simulink model "JointSpace_Task_v2"  (R2020b)
settings: Solver=ode3  StartTime=0.0  StopTime=6  FixedStep=0.05  RelTol=1e-3
libraries: XBotBlockToolbox x1, simulink x1, Utilities x1

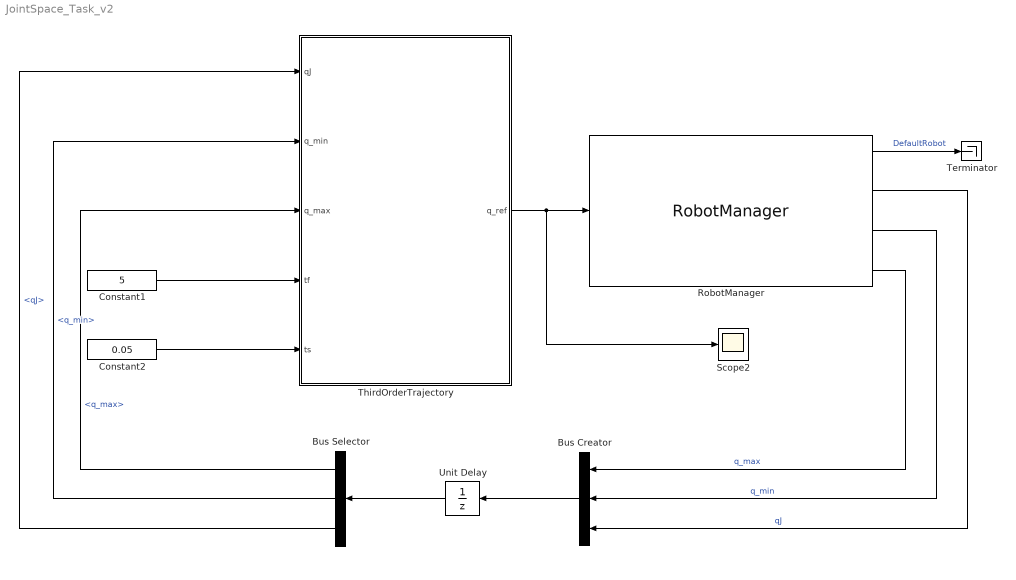
== system JointSpace_Task_v2 ==
  Bus Creator : BusCreator  Inputs=3
  Bus Selector : BusSelector  OutputSignals=q_max,q_min,qJ
  Constant1 : Constant  Value=5
  Constant2 : Constant  Value=0.05
  RobotManager : XBotBlockToolbox/RobotManager  RobotName=DefaultRobot  ModelName=DefaultModel  UseExtRobot=Off  SyncWithModel=Off  ReadingsList={ 'qJ' }  MechanicalLimitsList={ 'q_min', 'q_max' }  MechanicalLimitsCheck=Off  MechanicalLimitsEnforce=Off  SensorList={}  ReferencesList={ 'qJ_ref' }  OldRobotName=DefaultRobot
  Scope2 : Scope
  Terminator : Terminator
  ThirdOrderTrajectory : Subsystem
  Unit Delay : UnitDelay  SampleTime=-1  HasFrameUpgradeWarning=on
  wires:
  Constant1/1 -> ThirdOrderTrajectory/4(tf)
  Constant2/1 -> ThirdOrderTrajectory/5(ts)
  RobotManager/1 -> Terminator/1  "DefaultRobot"
  ThirdOrderTrajectory/1(q_ref) -> Scope2/1, RobotManager/1
  RobotManager/3 -> Bus Creator/2  "q_min"
  RobotManager/4 -> Bus Creator/1  "q_max"
  Bus Creator/1 -> Unit Delay/1
  Unit Delay/1 -> Bus Selector/1
  Bus Selector/1 -> ThirdOrderTrajectory/3(q_max)  "<q_max>"
  Bus Selector/2 -> ThirdOrderTrajectory/2(q_min)  "<q_min>"
  Bus Selector/3 -> ThirdOrderTrajectory/1(qJ)  "<qJ>"
  RobotManager/2 -> Bus Creator/3  "qJ"

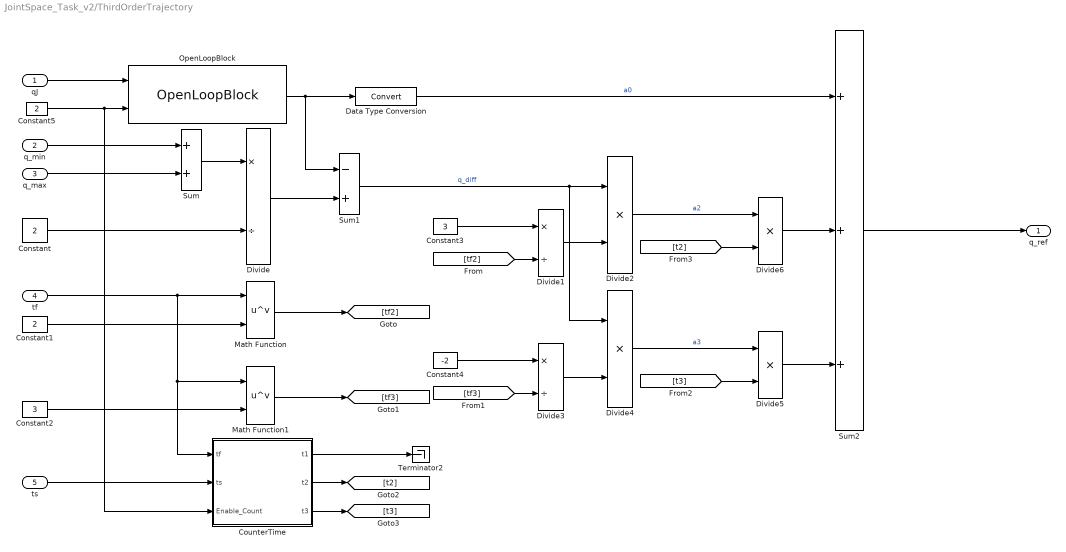
== system JointSpace_Task_v2/ThirdOrderTrajectory ==
  qJ : Inport
  q_min : Inport  Port=2
  q_max : Inport  Port=3
  tf : Inport  Port=4
  ts : Inport  Port=5
  Constant : Constant  Value=2
  Constant1 : Constant  Value=2
  Constant2 : Constant  Value=3
  Constant3 : Constant  Value=3
  Constant4 : Constant  Value=-2
  Constant5 : Constant  Value=2
  CounterTime : Subsystem
  Data Type Conversion : DataTypeConversion
  Divide : Product  Inputs=*/
  Divide1 : Product  Inputs=*/
  Divide{2,4..6} (4 alike) : Product  Inputs=**
  Divide3 : Product  Inputs=*/
  Math Function : Math  Operator=pow  SaturateOnIntegerOverflow=on
  Math Function1 : Math  Operator=pow  SaturateOnIntegerOverflow=on
  OpenLoopBlock : Utilities/OpenLoopBlock  SystemSampleTime=-1  VariantActivationTime=update diagram  Latency=0  AutoFrameSizeCalculation=off
  Sum : Sum
  Sum1 : Sum  Inputs=-+
  Sum2 : Sum  Inputs=+++
  Terminator2 : Terminator
  q_ref : Outport
  wires:
  q_min/1 -> Sum/1
  q_max/1 -> Sum/2
  Sum/1 -> Divide/1
  Constant/1 -> Divide/2
  tf/1 -> CounterTime/1(tf), Math Function1/1, Math Function/1
  Constant1/1 -> Math Function/2
  Constant2/1 -> Math Function1/2
  ts/1 -> CounterTime/2(ts)
  OpenLoopBlock/1 -> Sum1/1, Data Type Conversion/1
  Sum2/1 -> q_ref/1
  Math Function1/1 -> [tf3]
  Math Function/1 -> [tf2]
  CounterTime/1(t1) -> Terminator2/1
  CounterTime/2(t2) -> [t2]
  CounterTime/3(t3) -> [t3]
  Sum1/1 -> Divide4/1, Divide2/1  "q_diff"
  [tf2] -> Divide1/2
  Constant3/1 -> Divide1/1
  Divide1/1 -> Divide2/2
  Constant4/1 -> Divide3/1
  Divide3/1 -> Divide4/2
  [tf3] -> Divide3/2
  Divide2/1 -> Divide6/1  "a2"
  Divide4/1 -> Divide5/1  "a3"
  [t3] -> Divide5/2
  [t2] -> Divide6/2
  Data Type Conversion/1 -> Sum2/1  "a0"
  Divide6/1 -> Sum2/2
  Divide5/1 -> Sum2/3
  Divide/1 -> Sum1/2
  Constant5/1 -> CounterTime/3(Enable_Count), OpenLoopBlock/2
  qJ/1 -> OpenLoopBlock/1

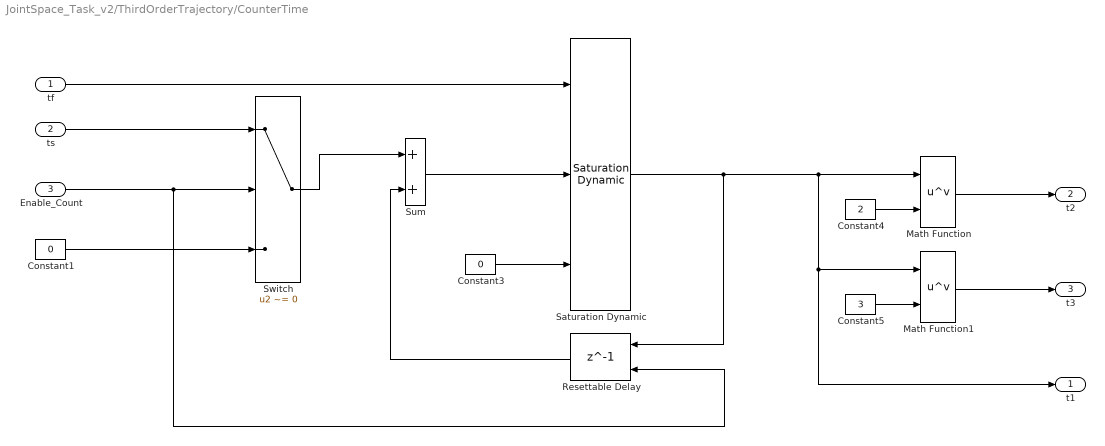
== system JointSpace_Task_v2/ThirdOrderTrajectory/CounterTime ==
  tf : Inport
  ts : Inport  Port=2
  Enable_Count : Inport  Port=3
  Constant1 : Constant  Value=0
  Constant3 : Constant  Value=0
  Constant4 : Constant  Value=2
  Constant5 : Constant  Value=3
  Math Function : Math  Operator=pow  SaturateOnIntegerOverflow=on
  Math Function1 : Math  Operator=pow  SaturateOnIntegerOverflow=on
  Resettable Delay : Delay  DelayLength=1  ExternalReset=Rising
  Saturation Dynamic : simulink/Discontinuities/Saturation Dynamic  OutMin=[]  OutMax=[]  OutDataTypeStr=Inherit: Same as second input  OutDataType=fixdt(1, 16)  OutScaling=2^-10  DoSatur=off
  Sum : Sum
  Switch : Switch  Criteria=u2 ~= 0
  t1 : Outport
  t2 : Outport  Port=2
  t3 : Outport  Port=3
  wires:
  Constant3/1 -> Saturation Dynamic/3
  Saturation Dynamic/1 -> Resettable Delay/1, t1/1, Math Function1/1, Math Function/1
  tf/1 -> Saturation Dynamic/1
  ts/1 -> Switch/1
  Sum/1 -> Saturation Dynamic/2
  Resettable Delay/1 -> Sum/2
  Switch/1 -> Sum/1
  Constant1/1 -> Switch/3
  Constant4/1 -> Math Function/2
  Constant5/1 -> Math Function1/2
  Math Function/1 -> t2/1
  Math Function1/1 -> t3/1
  Enable_Count/1 -> Resettable Delay/2, Switch/2
